simulink model "Starter_harness"  (Simulink 7.7)
settings: Solver=FixedStepDiscrete  SolverMode=SingleTasking  StartTime=0.0  StopTime=100  FixedStep=0.01  RelTol=1e-3
InitFcn:
  | if signalbuilder('Starter_harness/Signal_Builder','activegroup') == 10
  |   CD_STARTER_DEBOUNCE_NORMAL.DataType = 'uint16';
  |   CD_STARTER_DEBOUNCE_NORMAL.Value = 65535;
  | else
  |   CD_STARTER_DEBOUNCE_NORMAL.DataType = 'uint16';
  |   CD_STARTER_DEBOUNCE_NORMAL.Value = 300;
  | end
  | 
  | if signalbuilder('Starter_harness/Signal_Builder','activegroup') == 11
  |   CD_STARTER_FUNCTION.DataType = 'uint8';
  |   CD_STARTER_FUNCTION.Value = 255;
  | else
  |   CD_STARTER_FUNCTION.DataType = 'uint8';
  |   CD_STARTER_FUNCTION.Value = 0;
  | end
  | 
  | if signalbuilder('Starter_harness/Signal_Builder','activegroup') == 12
  |   CD_STARTER_FEEDBACK_FUNCTION.DataType = 'uint8';
  |   CD_STARTER_FEEDBACK_FUNCTION.Value = 255;
  | else
  |   CD_STARTER_FEEDBACK_FUNCTION.DataType = 'uint8';
  |   CD_STARTER_FEEDBACK_FUNCTION.Value = 0;
  | end
undefined symbols (not defined in the file): ACTIVE, ENGINE_CRANKING, ERROR_ON, INACTIVE, NON_FUNCTIONAL, NORMAL, OORL, sigbuilder_block, srate
libraries: simulink x2, MX_Library x1
CloseFcn:
  | rtwprivate ssgencode ModelCloseRequest sle_main_controller
settings Model: Creator=smindema  LastModifiedBy=aliebel  RecordCoverage=on  CovPath=Starter  CovMetricSettings=dcmw  CovHTMLOptions=-aTS=1 -bRG=1 -bTC=1 -hTR=0 -nFC=0 -scm=1 -bcm=1 -xEv=0  CovForceBlockReductionOff=off  covSaveCumulativeToWorkspaceVar=off  CovModelRefEnable=off
settings MATStruct: SampleTime=0.01  Offset=0  Priority=[1.0]
settings DataIOCC: LimitDataPoints=off  SaveOutput=off  SaveTime=off
settings OptimizationCC: BlockReduction=off  InlineParams=on  ExpressionFolding=off  StateBitsets=on  DataBitsets=on  UseTempVars=on  InitFltsAndDblsToZero=on  NoFixptDivByZeroProtection=on  EfficientFloat2IntCast=on  OptimizeModelRefInitCode=on
settings DebuggingCC: SaveWithParameterizedLinksMsg=none  MultiTaskDSMMsg=warning  MultiTaskCondExecSysMsg=none  IntegerOverflowMsg=none  ModelReferenceCSMismatchMessage=warning
settings HardwareCC: ProdBitPerInt=16  ProdBitPerPointer=16  ProdIntDivRoundTo=Floor  ProdEndianess=BigEndian  ProdWordSize=16  ProdHWDeviceType=Motorola HC12
settings ModelReferenceCC: ModelReferenceNumInstancesAllowed=Single
settings RTWCC: SystemTargetFile=ert.tlc  GenCodeOnly=on  TemplateMakefile=ert_default_tmf  Description=Real-Time Workshop Embedded Coder (no auto configuration)  GenerateReport=on  RetainRTWFile=on  ProcessScript=ert_make_rtw_hook  IncludeHyperlinkInReport=on  LaunchReport=on  IncludeERTFirstTime=on
settings RTWCC: CustomHeaderCode=|
  | #include "cpp_req_defines.h"
  | #include "hw_fin.h"
  | #include "cdata.h"
settings CodeAppCC: IgnoreCustomStorageClasses=off  DefineNamingRule=UpperCase
settings ERTTargetCC: TargetFcnLib=ansi_tfl_tmw.mat  FunctionExecutionProfile=off  MultiwordLength=2048  GenerateSampleERTMain=on  IncludeMdlTerminateFcn=off  SupportAbsoluteTime=off  SupportNonFinite=off  SupportComplex=off  PurelyIntegerCode=on  ERTCustomFileTemplate=gen_rtw_req_defines_h.tlc  GlobalDataDefinition=InSeparateSourceFile  GlobalDataReference=InSeparateHeaderFile  ConvertIfToSwitch=off

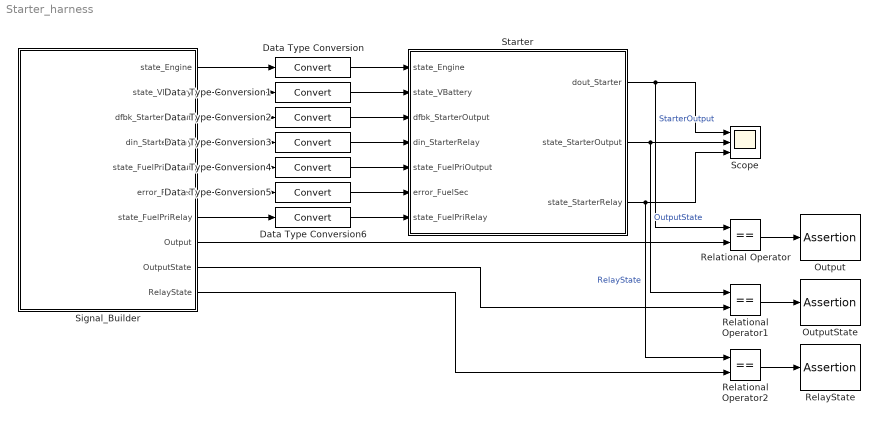
== system Starter_harness ==
  Data Type Conversion{,1..6} (7 alike) : DataTypeConversion
  Output : Assertion  Enabled=off
  OutputState : Assertion  Enabled=off
  Relational Operator : RelationalOperator  Operator===  OutDataTypeStr=boolean
  Relational Operator1 : RelationalOperator  Operator===  OutDataTypeStr=boolean
  Relational Operator2 : RelationalOperator  Operator===  OutDataTypeStr=boolean
  RelayState : Assertion  Enabled=off
  Scope : Scope  NumInputPorts=3
      settings: TimeRange=100  YMin=0~0~0  YMax=1~28~10  MaxDataPoints=50000
  Signal_Builder : Subsystem  Tag=STV Subsys  LoadFcn=sigbuilder_block('load',[285 55.5 1080 603.75 ]);  StartFcn=sigbuilder_block('start');  StopFcn=sigbuilder_block('stop');  ClipboardFcn=sigbuilder_block('clipboard');  mask(Sigbuilder block){}
      mask help: Sigbuilder GUI
      mask init:
      | if ~strcmp(get_param(bdroot(gcbh),'SimulationStatus'),'stopped') tuvar = sigbuilder_block('maskInit'); end
      settings: CopyFcn=sigbuilder_block('copy');  DeleteFcn=sigbuilder_block('delete');  ModelCloseFcn=sigbuilder_block('modelClose');  PreSaveFcn=sigbuilder_block('preSave');  NameChangeFcn=sigbuilder_block('namechange');  OpenFcn=sigbuilder_block('open',[0 21 1080 603.75 ]);  CloseFcn=sigbuilder_block('close');
      mask Display: plot(0,0,100,100,[10,10,40,40,10],[80,20,20,80,80],[40,10],[50,50], [40,27,10],[65,72,56],[40,25,25,10],[28,28,43,43]);
  Starter : Subsystem  TreatAsAtomicUnit=on  SystemSampleTime=srate  RTWFileName=mod_Outputs
      settings: RTWSystemCode=Function  RTWFileNameOpts=User specified
  wires:
  Starter/1(dout_Starter) -> Scope/1, Relational Operator/1  "StarterOutput"
  Starter/2(state_StarterOutput) -> Scope/2, Relational Operator1/1  "OutputState"
  Starter/3(state_StarterRelay) -> Scope/3, Relational Operator2/1  "RelayState"
  Data Type Conversion/1 -> Starter/1(state_Engine)
  Data Type Conversion1/1 -> Starter/2(state_VBattery)
  Data Type Conversion2/1 -> Starter/3(dfbk_StarterOutput)
  Data Type Conversion3/1 -> Starter/4(din_StarterRelay)
  Data Type Conversion4/1 -> Starter/5(state_FuelPriOutput)
  Data Type Conversion5/1 -> Starter/6(error_FuelSec)
  Data Type Conversion6/1 -> Starter/7(state_FuelPriRelay)
  Relational Operator/1 -> Output/1
  Relational Operator1/1 -> OutputState/1
  Relational Operator2/1 -> RelayState/1
  Signal_Builder/8(Output) -> Relational Operator/2
  Signal_Builder/9(OutputState) -> Relational Operator1/2
  Signal_Builder/10(RelayState) -> Relational Operator2/2
  Signal_Builder/1(state_Engine) -> Data Type Conversion/1
  Signal_Builder/2(state_VBattery) -> Data Type Conversion1/1
  Signal_Builder/3(dfbk_StarterOutput) -> Data Type Conversion2/1
  Signal_Builder/4(din_StarterRelay) -> Data Type Conversion3/1
  Signal_Builder/5(state_FuelPriOutput) -> Data Type Conversion4/1
  Signal_Builder/6(error_FuelSec) -> Data Type Conversion5/1
  Signal_Builder/7(state_FuelPriRelay) -> Data Type Conversion6/1

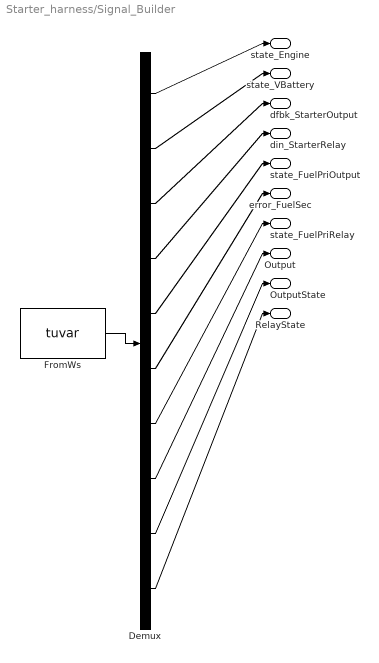
== system Starter_harness/Signal_Builder ==
  Demux : Demux  Tag=STV Demux  Outputs=10
  FromWs : FromWorkspace  Tag=STV FromWs  VariableName=tuvar  SampleTime=0  SigBuilderData=DataTag0  VnvData=DataTag1
      SigBuilderData=|
      | common.afterFinalStr = 'Extrapolate'
      | common.sampleTime = 0
      | dataSet(1).timeRange = [0 100]
      | dataSet(1).name = 'Normal'
      | dataSet(2).timeRange = [0 100]
      | dataSet(2).name = 'Batt OORL'
      | dataSet(3).timeRange = [0 100]
      | dataSet(3).name = 'FuelSolenoid'
      | dataSet(4).timeRange = [0 100]
      | dataSet(4).name = 'Error OFF'
      | dataSet(5).timeRange = [0 100]
      | dataSet(5).name = 'Error ON'
      | dataSet(6).timeRange = [0 100]
      | dataSet(6).name = 'Controller Failure'
      | dataSet(7).timeRange = [0 100]
      | dataSet(7).name = 'Open circuit1'
      | dataSet(8).timeRange = [0 100]
      | dataSet(8).name = 'OC2'
      | dataSet(9).timeRange = [0 100]
      | dataSet(9).name = 'Relay EON'
      | dataSet(10).timeRange = [0 100]
      | dataSet(10).name = 'Error OFF Unlimited'
      | dataSet(11).timeRange = [0 100]
      | dataSet(11).name = 'NONFUNC'
      | dataSet(12).timeRange = [0 100]
      | dataSet(12).name = 'FDBKOFF'
      | sbobj.Groups(1).Name = 'Normal'
      | sbobj.Groups(1).Signals(1).Name = 'state_Engine'
      | sbobj.Groups(1).Signals(1).XData = [0 20 20 50 50 80 80 100]
      | sbobj.Groups(1).Signals(1).YData = [1 1 2 2 3 3 1 1]
      | sbobj.Groups(1).Signals(2).Name = 'state_VBattery'
      | sbobj.Groups(1).Signals(2).XData = [0 100]
      | sbobj.Groups(1).Signals(2).YData = [8 8]
      | sbobj.Groups(1).Signals(3).Name = 'dfbk_StarterOutput'
      | sbobj.Groups(1).Signals(3).XData = [0 20.2 20.2 50 50 100]
      | sbobj.Groups(1).Signals(3).YData = [0 0 1 1 0 0]
      | sbobj.Groups(1).Signals(4).Name = 'din_StarterRelay'
      | sbobj.Groups(1).Signals(4).XData = [0 20 20 50 50 100]
      | sbobj.Groups(1).Signals(4).YData = [0 0 1 1 0 0]
      | sbobj.Groups(1).Signals(5).Name = 'state_FuelPriOutput'
      | sbobj.Groups(1).Signals(5).XData = [0 100]
      | sbobj.Groups(1).Signals(5).YData = [8 8]
      | sbobj.Groups(1).Signals(6).Name = 'error_FuelSec'
      | sbobj.Groups(1).Signals(6).XData = [0 100]
      | sbobj.Groups(1).Signals(6).YData = [8 8]
      | sbobj.Groups(1).Signals(7).Name = 'state_FuelPriRelay'
      | sbobj.Groups(1).Signals(7).XData = [0 100]
      | sbobj.Groups(1).Signals(7).YData = [8 8]
      | sbobj.Groups(1).Signals(8).Name = 'Output'
      | sbobj.Groups(1).Signals(8).XData = [0 20 20 50 50 100]
      | sbobj.Groups(1).Signals(8).YData = [0 0 1 1 0 0]
      | sbobj.Groups(1).Signals(9).Name = 'OutputState'
      | sbobj.Groups(1).Signals(9).XData = [0 100]
      | sbobj.Groups(1).Signals(9).YData = [8 8]
      | sbobj.Groups(1).Signals(10).Name = 'RelayState'
      | sbobj.Groups(1).Signals(10).XData = [0 100]
      | sbobj.Groups(1).Signals(10).YData = [8 8]
      | sbobj.Groups(2).Name = 'Batt OORL'
      | sbobj.Groups(2).Signals(1).Name = 'state_Engine'
      | sbobj.Groups(2).Signals(1).XData = [0 20 20 50 50 80 80 100]
      | sbobj.Groups(2).Signals(1).YData = [1 1 2 2 3 3 1 1]
      | sbobj.Groups(2).Signals(2).Name = 'state_VBattery'
      | sbobj.Groups(2).Signals(2).XData = [0 16.6 16.6 24 24 41 41 47.8 47.8 100]
      | sbobj.Groups(2).Signals(2).YData = [8 8 22 22 8 8 22 22 8 8]
      | sbobj.Groups(2).Signals(3).Name = 'dfbk_StarterOutput'
      | sbobj.Groups(2).Signals(3).XData = [0 24 24 41 41 48 48 50 50 100]
      | sbobj.Groups(2).Signals(3).YData = [0 0 1 1 0 0 1 1 0 0]
      | sbobj.Groups(2).Signals(4).Name = 'din_StarterRelay'
      | sbobj.Groups(2).Signals(4).XData = [0 24 24 41 41 48 48 50 50 100]
      | sbobj.Groups(2).Signals(4).YData = [0 0 1 1 0 0 1 1 0 0]
      | sbobj.Groups(2).Signals(5).Name = 'state_FuelPriOutput'
      | sbobj.Groups(2).Signals(5).XData = [0 100]
      | sbobj.Groups(2).Signals(5).YData = [8 8]
      | sbobj.Groups(2).Signals(6).Name = 'error_FuelSec'
      | sbobj.Groups(2).Signals(6).XData = [0 100]
      | sbobj.Groups(2).Signals(6).YData = [8 8]
      | sbobj.Groups(2).Signals(7).Name = 'state_FuelPriRelay'
      | sbobj.Groups(2).Signals(7).XData = [0 100]
      | sbobj.Groups(2).Signals(7).YData = [8 8]
      | sbobj.Groups(2).Signals(8).Name = 'Output'
      | sbobj.Groups(2).Signals(8).XData = [0 24 24 41 41 47.8 47.8 50 50 100]
      | sbobj.Groups(2).Signals(8).YData = [0 0 1 1 0 0 1 1 0 0]
      | sbobj.Groups(2).Signals(9).Name = 'OutputState'
      | sbobj.Groups(2).Signals(9).XData = [0 100]
      | sbobj.Groups(2).Signals(9).YData = [8 8]
      | sbobj.Groups(2).Signals(10).Name = 'RelayState'
      | sbobj.Groups(2).Signals(10).XData = [0 100]
      | sbobj.Groups(2).Signals(10).YData = [8 8]
      | sbobj.Groups(3).Name = 'FuelSolenoid'
      | sbobj.Groups(3).Signals(1).Name = 'state_Engine'
      | sbobj.Groups(3).Signals(1).XData = [0 20 20 50 80 80 100]
      | sbobj.Groups(3).Signals(1).YData = [1 1 2 2 2 1 1]
      | sbobj.Groups(3).Signals(2).Name = 'state_VBattery'
      | sbobj.Groups(3).Signals(2).XData = [0 100]
      | sbobj.Groups(3).Signals(2).YData = [8 8]
      | sbobj.Groups(3).Signals(3).Name = 'dfbk_StarterOutput'
      | sbobj.Groups(3).Signals(3).XData = [0 20 30 30 40 40 50 50 60 60 70 70 80 80 100]
      | sbobj.Groups(3).Signals(3).YData = [0 0 0 1 1 0 0 1 1 0 0 1 1 0 0]
      | sbobj.Groups(3).Signals(4).Name = 'din_StarterRelay'
      | sbobj.Groups(3).Signals(4).XData = [0 20 30 30 40 40 50 50 60 60 70 70 80 80 100]
      | sbobj.Groups(3).Signals(4).YData = [0 0 0 1 1 0 0 1 1 0 0 1 1 0 0]
      | sbobj.Groups(3).Signals(5).Name = 'state_FuelPriOutput'
      | sbobj.Groups(3).Signals(5).XData = [0 60 60 70 70 100]
      | sbobj.Groups(3).Signals(5).YData = [8 8 7 7 8 8]
      | sbobj.Groups(3).Signals(6).Name = 'error_FuelSec'
      | sbobj.Groups(3).Signals(6).XData = [0 20 20 24.2 24.2 25.3 25.3 30 30 100]
      | sbobj.Groups(3).Signals(6).YData = [8 8 5 5 8 8 5 5 8 8]
      | sbobj.Groups(3).Signals(7).Name = 'state_FuelPriRelay'
      | sbobj.Groups(3).Signals(7).XData = [0 40 40 50 50 100]
      | sbobj.Groups(3).Signals(7).YData = [8 8 9 9 8 8]
      | sbobj.Groups(3).Signals(8).Name = 'Output'
      | sbobj.Groups(3).Signals(8).XData = [0 24.21 24.21 25.3 25.3 30 30 40 40 50 50 60 60 70 70 80 80 100]
      | sbobj.Groups(3).Signals(8).YData = [0 0 1 1 0 0 1 1 0 0 1 1 0 0 1 1 0 0]
      | sbobj.Groups(3).Signals(9).Name = 'OutputState'
      | sbobj.Groups(3).Signals(9).XData = [0 100]
      | sbobj.Groups(3).Signals(9).YData = [8 8]
      | sbobj.Groups(3).Signals(10).Name = 'RelayState'
      | sbobj.Groups(3).Signals(10).XData = [0 100]
      | sbobj.Groups(3).Signals(10).YData = [8 8]
      | sbobj.Groups(4).Name = 'Error OFF'
      | sbobj.Groups(4).Signals(1).Name = 'state_Engine'
      | sbobj.Groups(4).Signals(1).XData = [0 20 20 50 50 80 80 100]
      | sbobj.Groups(4).Signals(1).YData = [1 1 2 2 3 3 1 1]
      | sbobj.Groups(4).Signals(2).Name = 'state_VBattery'
      | sbobj.Groups(4).Signals(2).XData = [0 100]
      | sbobj.Groups(4).Signals(2).YData = [8 8]
      | sbobj.Groups(4).Signals(3).Name = 'dfbk_StarterOutput'
      | sbobj.Groups(4).Signals(3).XData = [0 20.2 50 100]
      | sbobj.Groups(4).Signals(3).YData = [0 0 0 0]
      | sbobj.Groups(4).Signals(4).Name = 'din_StarterRelay'
      | sbobj.Groups(4).Signals(4).XData = [0 100]
      | sbobj.Groups(4).Signals(4).YData = [0 0]
      | sbobj.Groups(4).Signals(5).Name = 'state_FuelPriOutput'
      | sbobj.Groups(4).Signals(5).XData = [0 100]
      | sbobj.Groups(4).Signals(5).YData = [8 8]
      | sbobj.Groups(4).Signals(6).Name = 'error_FuelSec'
      | sbobj.Groups(4).Signals(6).XData = [0 100]
      | sbobj.Groups(4).Signals(6).YData = [8 8]
      | sbobj.Groups(4).Signals(7).Name = 'state_FuelPriRelay'
      | sbobj.Groups(4).Signals(7).XData = [0 100]
      | sbobj.Groups(4).Signals(7).YData = [8 8]
      | sbobj.Groups(4).Signals(8).Name = 'Output'
      | sbobj.Groups(4).Signals(8).XData = [0 20 20 50 50 100]
      | sbobj.Groups(4).Signals(8).YData = [0 0 1 1 0 0]
      | sbobj.Groups(4).Signals(9).Name = 'OutputState'
      | sbobj.Groups(4).Signals(9).XData = [0 23.01 23.01 53.01 53.01 100]
      | sbobj.Groups(4).Signals(9).YData = [8 8 3 3 8 8]
      | sbobj.Groups(4).Signals(10).Name = 'RelayState'
      | sbobj.Groups(4).Signals(10).XData = [0 23.01 53.01 100]
      | sbobj.Groups(4).Signals(10).YData = [8 8 8 8]
      | sbobj.Groups(5).Name = 'Error ON'
      | sbobj.Groups(5).Signals(1).Name = 'state_Engine'
      | sbobj.Groups(5).Signals(1).XData = [0 20 20 50 50 80 80 100]
      | sbobj.Groups(5).Signals(1).YData = [1 1 2 2 3 3 1 1]
      | sbobj.Groups(5).Signals(2).Name = 'state_VBattery'
      | sbobj.Groups(5).Signals(2).XData = [0 100]
      | sbobj.Groups(5).Signals(2).YData = [8 8]
      | sbobj.Groups(5).Signals(3).Name = 'dfbk_StarterOutput'
      | sbobj.Groups(5).Signals(3).XData = [0 10 10 20 20 26.01 26.01 50 50 100]
      | sbobj.Groups(5).Signals(3).YData = [0 0 1 1 0 0 1 1 0 0]
      | sbobj.Groups(5).Signals(4).Name = 'din_StarterRelay'
      | sbobj.Groups(5).Signals(4).XData = [0 10 10 20 20 26.01 26.01 49.8 49.8 100]
      | sbobj.Groups(5).Signals(4).YData = [0 0 1 1 0 0 1 1 0 0]
      | sbobj.Groups(5).Signals(5).Name = 'state_FuelPriOutput'
      | sbobj.Groups(5).Signals(5).XData = [0 100]
      | sbobj.Groups(5).Signals(5).YData = [8 8]
      | sbobj.Groups(5).Signals(6).Name = 'error_FuelSec'
      | sbobj.Groups(5).Signals(6).XData = [0 100]
      | sbobj.Groups(5).Signals(6).YData = [8 8]
      | sbobj.Groups(5).Signals(7).Name = 'state_FuelPriRelay'
      | sbobj.Groups(5).Signals(7).XData = [0 100]
      | sbobj.Groups(5).Signals(7).YData = [8 8]
      | sbobj.Groups(5).Signals(8).Name = 'Output'
      | sbobj.Groups(5).Signals(8).XData = [0 23.02 23.02 50 50 100]
      | sbobj.Groups(5).Signals(8).YData = [0 0 1 1 0 0]
      | sbobj.Groups(5).Signals(9).Name = 'OutputState'
      | sbobj.Groups(5).Signals(9).XData = [0 10.11 10.11 23.01 23.01 100]
      | sbobj.Groups(5).Signals(9).YData = [8 8 2 2 8 8]
      | sbobj.Groups(5).Signals(10).Name = 'RelayState'
      | sbobj.Groups(5).Signals(10).XData = [0 13.01 23.01 100]
      | sbobj.Groups(5).Signals(10).YData = [8 8 8 8]
      | sbobj.Groups(6).Name = 'Controller Failure'
      | sbobj.Groups(6).Signals(1).Name = 'state_Engine'
      | sbobj.Groups(6).Signals(1).XData = [0 20 20 50 50 80 80 100]
      | sbobj.Groups(6).Signals(1).YData = [1 1 2 2 3 3 1 1]
      | sbobj.Groups(6).Signals(2).Name = 'state_VBattery'
      | sbobj.Groups(6).Signals(2).XData = [0 100]
      | sbobj.Groups(6).Signals(2).YData = [8 8]
      | sbobj.Groups(6).Signals(3).Name = 'dfbk_StarterOutput'
      | sbobj.Groups(6).Signals(3).XData = [0 20.2 20.2 50 50 100]
      | sbobj.Groups(6).Signals(3).YData = [0 0 0 0 0 0]
      | sbobj.Groups(6).Signals(4).Name = 'din_StarterRelay'
      | sbobj.Groups(6).Signals(4).XData = [0 20 20 50 50 100]
      | sbobj.Groups(6).Signals(4).YData = [0 0 1 1 0 0]
      | sbobj.Groups(6).Signals(5).Name = 'state_FuelPriOutput'
      | sbobj.Groups(6).Signals(5).XData = [0 100]
      | sbobj.Groups(6).Signals(5).YData = [8 8]
      | sbobj.Groups(6).Signals(6).Name = 'error_FuelSec'
      | sbobj.Groups(6).Signals(6).XData = [0 100]
      | sbobj.Groups(6).Signals(6).YData = [8 8]
      | sbobj.Groups(6).Signals(7).Name = 'state_FuelPriRelay'
      | sbobj.Groups(6).Signals(7).XData = [0 100]
      | sbobj.Groups(6).Signals(7).YData = [8 8]
      | sbobj.Groups(6).Signals(8).Name = 'Output'
      | sbobj.Groups(6).Signals(8).XData = [0 20 20 50 50 100]
      | sbobj.Groups(6).Signals(8).YData = [0 0 1 1 0 0]
      | sbobj.Groups(6).Signals(9).Name = 'OutputState'
      | sbobj.Groups(6).Signals(9).XData = [0 23.01 23.01 53.01 53.01 100]
      | sbobj.Groups(6).Signals(9).YData = [8 8 28 28 8 8]
      | sbobj.Groups(6).Signals(10).Name = 'RelayState'
      | sbobj.Groups(6).Signals(10).XData = [0 100]
      | sbobj.Groups(6).Signals(10).YData = [8 8]
      | sbobj.Groups(7).Name = 'Open circuit1'
      | sbobj.Groups(7).Signals(1).Name = 'state_Engine'
      | sbobj.Groups(7).Signals(1).XData = [0 20 50 80 100]
      | sbobj.Groups(7).Signals(1).YData = [1 1 1 1 1]
      | sbobj.Groups(7).Signals(2).Name = 'state_VBattery'
      | sbobj.Groups(7).Signals(2).XData = [0 100]
      | sbobj.Groups(7).Signals(2).YData = [8 8]
      | sbobj.Groups(7).Signals(3).Name = 'dfbk_StarterOutput'
      | sbobj.Groups(7).Signals(3).XData = [0 10 10 43 43 50 100]
      | sbobj.Groups(7).Signals(3).YData = [0 0 1 1 0 0 0]
      | sbobj.Groups(7).Signals(4).Name = 'din_StarterRelay'
      | sbobj.Groups(7).Signals(4).XData = [0 20 50 100]
      | sbobj.Groups(7).Signals(4).YData = [0 0 0 0]
      | sbobj.Groups(7).Signals(5).Name = 'state_FuelPriOutput'
      | sbobj.Groups(7).Signals(5).XData = [0 100]
      | sbobj.Groups(7).Signals(5).YData = [8 8]
      | sbobj.Groups(7).Signals(6).Name = 'error_FuelSec'
      | sbobj.Groups(7).Signals(6).XData = [0 100]
      | sbobj.Groups(7).Signals(6).YData = [8 8]
      | sbobj.Groups(7).Signals(7).Name = 'state_FuelPriRelay'
      | sbobj.Groups(7).Signals(7).XData = [0 100]
      | sbobj.Groups(7).Signals(7).YData = [8 8]
      | sbobj.Groups(7).Signals(8).Name = 'Output'
      | sbobj.Groups(7).Signals(8).XData = [0 100]
      | sbobj.Groups(7).Signals(8).YData = [0 0]
      | sbobj.Groups(7).Signals(9).Name = 'OutputState'
      | sbobj.Groups(7).Signals(9).XData = [0 13.01 13.01 46.01 46.01 100]
      | sbobj.Groups(7).Signals(9).YData = [8 8 7 7 8 8]
      | sbobj.Groups(7).Signals(10).Name = 'RelayState'
      | sbobj.Groups(7).Signals(10).XData = [0 13.01 100]
      | sbobj.Groups(7).Signals(10).YData = [8 8 8]
      | sbobj.Groups(8).Name = 'OC2'
      | sbobj.Groups(8).Signals(1).Name = 'state_Engine'
      | sbobj.Groups(8).Signals(1).XData = [0 20 20 50 50 80 80 100]
      | sbobj.Groups(8).Signals(1).YData = [1 1 2 2 3 3 1 1]
      | sbobj.Groups(8).Signals(2).Name = 'state_VBattery'
      | sbobj.Groups(8).Signals(2).XData = [0 100]
      | sbobj.Groups(8).Signals(2).YData = [8 8]
      | sbobj.Groups(8).Signals(3).Name = 'dfbk_StarterOutput'
      | sbobj.Groups(8).Signals(3).XData = [0 20 20 50 50 100]
      | sbobj.Groups(8).Signals(3).YData = [0 0 1 1 0 0]
      | sbobj.Groups(8).Signals(4).Name = 'din_StarterRelay'
      | sbobj.Groups(8).Signals(4).XData = [0 20 50 100]
      | sbobj.Groups(8).Signals(4).YData = [0 0 0 0]
      | sbobj.Groups(8).Signals(5).Name = 'state_FuelPriOutput'
      | sbobj.Groups(8).Signals(5).XData = [0 100]
      | sbobj.Groups(8).Signals(5).YData = [8 8]
      | sbobj.Groups(8).Signals(6).Name = 'error_FuelSec'
      | sbobj.Groups(8).Signals(6).XData = [0 100]
      | sbobj.Groups(8).Signals(6).YData = [8 8]
      | sbobj.Groups(8).Signals(7).Name = 'state_FuelPriRelay'
      | sbobj.Groups(8).Signals(7).XData = [0 100]
      | sbobj.Groups(8).Signals(7).YData = [8 8]
      | sbobj.Groups(8).Signals(8).Name = 'Output'
      | sbobj.Groups(8).Signals(8).XData = [0 20 20 50 50 100]
      | sbobj.Groups(8).Signals(8).YData = [0 0 1 1 0 0]
      | sbobj.Groups(8).Signals(9).Name = 'OutputState'
      | sbobj.Groups(8).Signals(9).XData = [0 100]
      | sbobj.Groups(8).Signals(9).YData = [8 8]
      | sbobj.Groups(8).Signals(10).Name = 'RelayState'
      | sbobj.Groups(8).Signals(10).XData = [0 23.01 23.01 53.01 53.01 100]
      | sbobj.Groups(8).Signals(10).YData = [8 8 3 3 8 8]
      | sbobj.Groups(9).Name = 'Relay EON'
      | sbobj.Groups(9).Signals(1).Name = 'state_Engine'
      | sbobj.Groups(9).Signals(1).XData = [0 20 30 30 50 50 80 100]
      | sbobj.Groups(9).Signals(1).YData = [1 1 1 2 2 1 1 1]
      | sbobj.Groups(9).Signals(2).Name = 'state_VBattery'
      | sbobj.Groups(9).Signals(2).XData = [0 100]
      | sbobj.Groups(9).Signals(2).YData = [8 8]
      | sbobj.Groups(9).Signals(3).Name = 'dfbk_StarterOutput'
      | sbobj.Groups(9).Signals(3).XData = [0 10 42.6 50 100]
      | sbobj.Groups(9).Signals(3).YData = [0 0 0 0 0]
      | sbobj.Groups(9).Signals(4).Name = 'din_StarterRelay'
      | sbobj.Groups(9).Signals(4).XData = [0 20 20 50 50 100]
      | sbobj.Groups(9).Signals(4).YData = [0 0 1 1 0 0]
      | sbobj.Groups(9).Signals(5).Name = 'state_FuelPriOutput'
      | sbobj.Groups(9).Signals(5).XData = [0 100]
      | sbobj.Groups(9).Signals(5).YData = [8 8]
      | sbobj.Groups(9).Signals(6).Name = 'error_FuelSec'
      | sbobj.Groups(9).Signals(6).XData = [0 100]
      | sbobj.Groups(9).Signals(6).YData = [8 8]
      | sbobj.Groups(9).Signals(7).Name = 'state_FuelPriRelay'
      | sbobj.Groups(9).Signals(7).XData = [0 100]
      | sbobj.Groups(9).Signals(7).YData = [8 8]
      | sbobj.Groups(9).Signals(8).Name = 'Output'
      | sbobj.Groups(9).Signals(8).XData = [0 30 50 100]
      | sbobj.Groups(9).Signals(8).YData = [0 0 0 0]
      | sbobj.Groups(9).Signals(9).Name = 'OutputState'
      | sbobj.Groups(9).Signals(9).XData = [0 100]
      | sbobj.Groups(9).Signals(9).YData = [8 8]
      | sbobj.Groups(9).Signals(10).Name = 'RelayState'
      | sbobj.Groups(9).Signals(10).XData = [0 20.11 20.11 53.01 53.01 100]
      | sbobj.Groups(9).Signals(10).YData = [8 8 2 2 8 8]
      | sbobj.Groups(10).Name = 'Error OFF Unlimited'
      | sbobj.Groups(10).Signals(1).Name = 'state_Engine'
      | sbobj.Groups(10).Signals(1).XData = [0 20 20 50 50 80 80 100]
      | sbobj.Groups(10).Signals(1).YData = [1 1 2 2 3 3 1 1]
      | sbobj.Groups(10).Signals(2).Name = 'state_VBattery'
      | sbobj.Groups(10).Signals(2).XData = [0 100]
      | sbobj.Groups(10).Signals(2).YData = [8 8]
      | sbobj.Groups(10).Signals(3).Name = 'dfbk_StarterOutput'
      | sbobj.Groups(10).Signals(3).XData = [0 20.2 50 100]
      | sbobj.Groups(10).Signals(3).YData = [0 0 0 0]
      | sbobj.Groups(10).Signals(4).Name = 'din_StarterRelay'
      | sbobj.Groups(10).Signals(4).XData = [0 100]
      | sbobj.Groups(10).Signals(4).YData = [0 0]
      | sbobj.Groups(10).Signals(5).Name = 'state_FuelPriOutput'
      | sbobj.Groups(10).Signals(5).XData = [0 100]
      | sbobj.Groups(10).Signals(5).YData = [8 8]
      | sbobj.Groups(10).Signals(6).Name = 'error_FuelSec'
      | sbobj.Groups(10).Signals(6).XData = [0 100]
      | sbobj.Groups(10).Signals(6).YData = [8 8]
      | sbobj.Groups(10).Signals(7).Name = 'state_FuelPriRelay'
      | sbobj.Groups(10).Signals(7).XData = [0 100]
      | sbobj.Groups(10).Signals(7).YData = [8 8]
      | sbobj.Groups(10).Signals(8).Name = 'Output'
      | sbobj.Groups(10).Signals(8).XData = [0 20 20 50 50 100]
      | sbobj.Groups(10).Signals(8).YData = [0 0 1 1 0 0]
      | sbobj.Groups(10).Signals(9).Name = 'OutputState'
      | sbobj.Groups(10).Signals(9).XData = [0 23.01 23.01 53.01 100]
      | sbobj.Groups(10).Signals(9).YData = [8 8 3 3 3]
      | sbobj.Groups(10).Signals(10).Name = 'RelayState'
      | sbobj.Groups(10).Signals(10).XData = [0 23.01 53.01 100]
      | sbobj.Groups(10).Signals(10).YData = [8 8 8 8]
      | sbobj.Groups(11).Name = 'NONFUNC'
      | sbobj.Groups(11).Signals(1).Name = 'state_Engine'
      | sbobj.Groups(11).Signals(1).XData = [0 20 20 50 50 80 80 100]
      | sbobj.Groups(11).Signals(1).YData = [1 1 2 2 3 3 1 1]
      | sbobj.Groups(11).Signals(2).Name = 'state_VBattery'
      | sbobj.Groups(11).Signals(2).XData = [0 100]
      | sbobj.Groups(11).Signals(2).YData = [8 8]
      | sbobj.Groups(11).Signals(3).Name = 'dfbk_StarterOutput'
      | sbobj.Groups(11).Signals(3).XData = [0 20.2 100]
      | sbobj.Groups(11).Signals(3).YData = [0 0 0]
      | sbobj.Groups(11).Signals(4).Name = 'din_StarterRelay'
      | sbobj.Groups(11).Signals(4).XData = [0 20 100]
      | sbobj.Groups(11).Signals(4).YData = [0 0 0]
      | sbobj.Groups(11).Signals(5).Name = 'state_FuelPriOutput'
      | sbobj.Groups(11).Signals(5).XData = [0 100]
      | sbobj.Groups(11).Signals(5).YData = [8 8]
      | sbobj.Groups(11).Signals(6).Name = 'error_FuelSec'
      | sbobj.Groups(11).Signals(6).XData = [0 100]
      | sbobj.Groups(11).Signals(6).YData = [8 8]
      | sbobj.Groups(11).Signals(7).Name = 'state_FuelPriRelay'
      | sbobj.Groups(11).Signals(7).XData = [0 100]
      | sbobj.Groups(11).Signals(7).YData = [8 8]
      | sbobj.Groups(11).Signals(8).Name = 'Output'
      | sbobj.Groups(11).Signals(8).XData = [0 100]
      | sbobj.Groups(11).Signals(8).YData = [0 0]
      | sbobj.Groups(11).Signals(9).Name = 'OutputState'
      | sbobj.Groups(11).Signals(9).XData = [0 100]
      | sbobj.Groups(11).Signals(9).YData = [8 8]
      | sbobj.Groups(11).Signals(10).Name = 'RelayState'
      | sbobj.Groups(11).Signals(10).XData = [0 100]
      | sbobj.Groups(11).Signals(10).YData = [8 8]
      | sbobj.Groups(12).Name = 'FDBKOFF'
      | sbobj.Groups(12).Signals(1).Name = 'state_Engine'
      | sbobj.Groups(12).Signals(1).XData = [0 20 20 50 50 80 80 100]
      | sbobj.Groups(12).Signals(1).YData = [1 1 2 2 3 3 1 1]
      | sbobj.Groups(12).Signals(2).Name = 'state_VBattery'
      | sbobj.Groups(12).Signals(2).XData = [0 100]
      | sbobj.Groups(12).Signals(2).YData = [8 8]
      | sbobj.Groups(12).Signals(3).Name = 'dfbk_StarterOutput'
      | sbobj.Groups(12).Signals(3).XData = [0 10 10 20 20 26.01 26.01 50 50 100]
      | sbobj.Groups(12).Signals(3).YData = [0 0 1 1 0 0 1 1 0 0]
      | sbobj.Groups(12).Signals(4).Name = 'din_StarterRelay'
      | sbobj.Groups(12).Signals(4).XData = [0 10 10 20 20 26.01 26.01 49.8 49.8 100]
      | sbobj.Groups(12).Signals(4).YData = [0 0 1 1 0 0 1 1 0 0]
      | sbobj.Groups(12).Signals(5).Name = 'state_FuelPriOutput'
      | sbobj.Groups(12).Signals(5).XData = [0 100]
      | sbobj.Groups(12).Signals(5).YData = [8 8]
      | sbobj.Groups(12).Signals(6).Name = 'error_FuelSec'
      | sbobj.Groups(12).Signals(6).XData = [0 100]
      | sbobj.Groups(12).Signals(6).YData = [8 8]
      | sbobj.Groups(12).Signals(7).Name = 'state_FuelPriRelay'
      | sbobj.Groups(12).Signals(7).XData = [0 100]
      | sbobj.Groups(12).Signals(7).YData = [8 8]
      | sbobj.Groups(12).Signals(8).Name = 'Output'
      | sbobj.Groups(12).Signals(8).XData = [0 20 20 50 50 100]
      | sbobj.Groups(12).Signals(8).YData = [0 0 1 1 0 0]
      | sbobj.Groups(12).Signals(9).Name = 'OutputState'
      | sbobj.Groups(12).Signals(9).XData = [0 13.01 23.01 100]
      | sbobj.Groups(12).Signals(9).YData = [8 8 8 8]
      | sbobj.Groups(12).Signals(10).Name = 'RelayState'
      | sbobj.Groups(12).Signals(10).XData = [0 13.01 23.01 100]
      | sbobj.Groups(12).Signals(10).YData = [8 8 8 8]
  state_Engine : Outport  Tag=STV Outport
  state_VBattery : Outport  Tag=STV Outport  Port=2
  dfbk_StarterOutput : Outport  Tag=STV Outport  Port=3
  din_StarterRelay : Outport  Tag=STV Outport  Port=4
  state_FuelPriOutput : Outport  Tag=STV Outport  Port=5
  error_FuelSec : Outport  Tag=STV Outport  Port=6
  state_FuelPriRelay : Outport  Tag=STV Outport  Port=7
  Output : Outport  Tag=STV Outport  Port=8
  OutputState : Outport  Tag=STV Outport  Port=9
  RelayState : Outport  Tag=STV Outport  Port=10
  wires:
  FromWs/1 -> Demux/1
  Demux/1 -> state_Engine/1
  Demux/2 -> state_VBattery/1
  Demux/3 -> dfbk_StarterOutput/1
  Demux/4 -> din_StarterRelay/1
  Demux/5 -> state_FuelPriOutput/1
  Demux/6 -> error_FuelSec/1
  Demux/7 -> state_FuelPriRelay/1
  Demux/8 -> Output/1
  Demux/9 -> OutputState/1
  Demux/10 -> RelayState/1

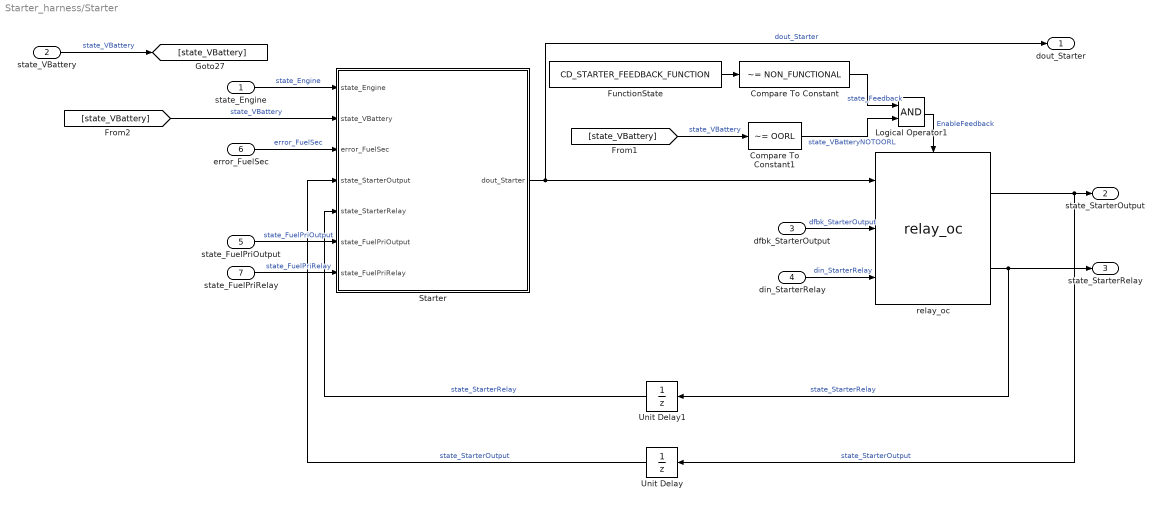
== system Starter_harness/Starter ==
  state_Engine : Inport
  state_VBattery : Inport  Port=2
  dfbk_StarterOutput : Inport  Port=3
  din_StarterRelay : Inport  Port=4
  state_FuelPriOutput : Inport  Port=5  OutDataTypeStr=uint8
  error_FuelSec : Inport  Port=6  OutDataTypeStr=uint8
  state_FuelPriRelay : Inport  Port=7  OutDataTypeStr=uint8
  Compare To Constant : simulink/Logic and Bit Operations/Compare To Constant  SystemSampleTime=-1  relop=~=  const=NON_FUNCTIONAL  LogicOutDataTypeMode=boolean  ZeroCross=off
  Compare To Constant1 : simulink/Logic and Bit Operations/Compare To Constant  SystemSampleTime=-1  relop=~=  const=OORL  LogicOutDataTypeMode=boolean  ZeroCross=off
  FunctionState : Constant  Value=CD_STARTER_FEEDBACK_FUNCTION  OutDataTypeStr=uint8
  Logical Operator1 : Logic  AllPortsSameDT=off  OutDataTypeStr=boolean
  Starter : Stateflow chart  TreatAsAtomicUnit=on
  Unit Delay : UnitDelay  X0=8  SampleTime=-1
      settings: AttributesFormatString=Initial Ouput = %<X0>
  Unit Delay1 : UnitDelay  X0=8  SampleTime=-1
      settings: AttributesFormatString=Initial Ouput = %<X0>
  relay_oc : MX_Library/relay_oc  SystemSampleTime=-1  ERROR_ON_DB_CNT=CD_STARTER_DEBOUNCE_ERROR_ON  ERROR_OFF_DB_CNT=CD_STARTER_DEBOUNCE_ERROR_OFF  NORMAL_DB_CNT=CD_STARTER_DEBOUNCE_NORMAL
  dout_Starter : Outport  OutDataTypeStr=boolean
  state_StarterOutput : Outport  Port=2  OutDataTypeStr=uint8
  state_StarterRelay : Outport  Port=3  OutDataTypeStr=uint8
  wires:
  Unit Delay1/1 -> Starter/5(state_StarterRelay)  "state_StarterRelay"
  Unit Delay/1 -> Starter/4(state_StarterOutput)  "state_StarterOutput"
  state_FuelPriRelay/1 -> Starter/7(state_FuelPriRelay)  "state_FuelPriRelay"
  state_VBattery/1 -> [state_VBattery]  "state_VBattery"
  Logical Operator1/1 -> relay_oc/Enable  "EnableFeedback"
  Compare To Constant1/1 -> Logical Operator1/2  "state_VBatteryNOTOORL"
  Compare To Constant/1 -> Logical Operator1/1  "state_Feedback"
  [state_VBattery] -> Compare To Constant1/1  "state_VBattery"
  FunctionState/1 -> Compare To Constant/1
  relay_oc/2 -> Unit Delay1/1, state_StarterRelay/1  "state_StarterRelay"
  relay_oc/1 -> Unit Delay/1, state_StarterOutput/1  "state_StarterOutput"
  din_StarterRelay/1 -> relay_oc/3  "din_StarterRelay"
  dfbk_StarterOutput/1 -> relay_oc/2  "dfbk_StarterOutput"
  error_FuelSec/1 -> Starter/3(error_FuelSec)  "error_FuelSec"
  state_FuelPriOutput/1 -> Starter/6(state_FuelPriOutput)  "state_FuelPriOutput"
  Starter/1(dout_Starter) -> dout_Starter/1, relay_oc/1  "dout_Starter"
  state_Engine/1 -> Starter/1(state_Engine)  "state_Engine"
  [state_VBattery] -> Starter/2(state_VBattery)  "state_VBattery"

== stateflow chart Starter/Starter ==
  state INACTIVE
    en:dout_Starter = INACTIVE;
  state ACTIVE
    en:dout_Starter = ACTIVE
  (default) -> INACTIVE
  INACTIVE -> ACTIVE : [(CD_STARTER_FUNCTION != NON_FUNCTIONAL)...
      | && (state_Engine == ENGINE_CRANKING)...
      | && (state_VBattery != OORL)...
      | && (state_StarterOutput != ERROR_ON)...
      | && (state_StarterRelay != ERROR_ON)...
      | && (error_FuelSec == NORMAL)...
      | && (state_FuelPriOutput == NORMAL)...
      | && (state_FuelPriRelay == NORMAL)]
  ACTIVE -> INACTIVE : [(state_Engine != ENGINE_CRANKING)...
      | || (state_VBattery == OORL)...
      | || (error_FuelSec != NORMAL)...
      | || (state_FuelPriOutput != NORMAL)...
      | || (state_FuelPriRelay != NORMAL)]
  data: state_Engine input uint8; state_VBattery input uint8; dout_Starter output boolean; CD_STARTER_FUNCTION parameter uint8; error_FuelSec input uint8; ACTIVE parameter uint8 =1; ENGINE_CRANKING parameter uint8 =2; INACTIVE parameter uint8 =0; NORMAL parameter uint8 =8; OORL parameter uint8 =22; NON_FUNCTIONAL parameter uint8 =255; state_StarterOutput input uint8; state_StarterRelay input uint8; ERROR_ON parameter uint8; state_FuelPriOutput input uint8; state_FuelPriRelay input uint8
